simulink model "bio_matfunc_fcn"  (R2017b)
settings: Solver=VariableStepAuto  StartTime=0.0  StopTime=10.0  RelTol=1e-3
settings Model: Creator=ktrinh  LastModifiedBy=ktrinh

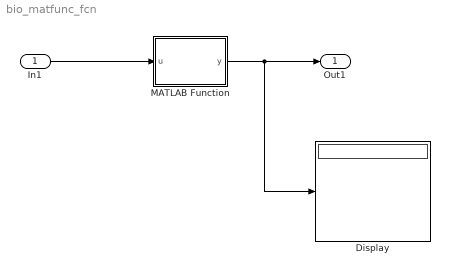
== system bio_matfunc_fcn ==
  In1 : Inport  OutDataTypeStr=double  PortDimensions=3
  Display : Display
  MATLAB Function : MATLAB Function  TreatAsAtomicUnit=on
  Out1 : Outport
  wires:
  In1/1 -> MATLAB Function/1(u)
  MATLAB Function/1(y) -> Display/1, Out1/1

== matlab function bio_matfunc_fcn/MATLAB Function ==
  data: u input; y output
function y = fcn(u)
%#codegen

y = u/norm(u);
